simulink model "Drivetrain_Bicycle"  (R2020a)
settings: Solver=VariableStepAuto  StartTime=0.0  StopTime=10.0  RelTol=1e-3
settings Model: Creator=yafta  LastModifiedBy=yafta

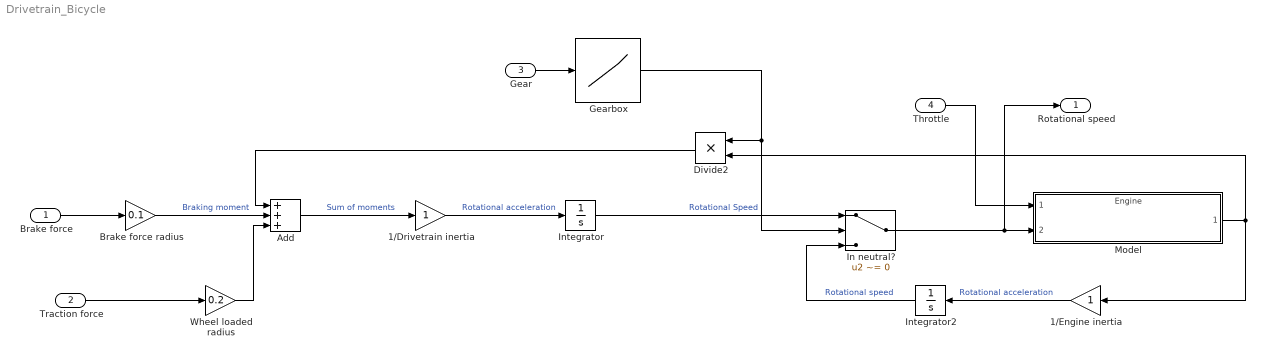
== system Drivetrain_Bicycle ==
  Brake force : Inport  OutDataTypeStr=double
  Traction force : Inport  Port=2  OutDataTypeStr=double
  Gear : Inport  Port=3  OutDataTypeStr=int8
  Throttle : Inport  Port=4  OutDataTypeStr=double
  1/Drivetrain inertia : Gain
  1/Engine inertia : Gain
  Add : Sum  Inputs=3
  Brake force radius : Gain  Gain=0.1
  Divide2 : Product  Inputs=**
  Gearbox : Lookup_n-D  NumberOfTableDimensions=1  BreakpointsForDimension1=[0,1,2,3,4,5,6]  BreakpointsForDimension1DataTypeStr=int8  Table=[0,2.583,2,1.667,1.444,1.286,1.15]  TableMin=0  TableMax=5  TableDataTypeStr=double  InterpMethod=Flat  DiagnosticForOutOfRangeInput=Error  InternalRulePriority=Speed  OutDataTypeStr=double  RndMeth=Simplest  InputSameDT=on
  In neutral? : Switch  Criteria=u2 ~= 0
  Integrator : Integrator
  Integrator2 : Integrator
  Model : ModelReference  ModelNameDialog=Engine  SimulationMode=Normal  ModelReferenceVersion=1.2
  Wheel loaded radius : Gain  Gain=0.2
  Rotational speed : Outport  OutDataTypeStr=double
  wires:
  1/Engine inertia/1 -> Integrator2/1  "Rotational acceleration"
  Traction force/1 -> Wheel loaded radius/1
  Integrator2/1 -> In neutral?/3  "Rotational speed"
  In neutral?/1 -> Model/2, Rotational speed/1
  Divide2/1 -> Add/1
  Integrator/1 -> In neutral?/1  "Rotational Speed"
  Brake force radius/1 -> Add/2  "Braking moment"
  Add/1 -> 1/Drivetrain inertia/1  "Sum of moments"
  Gearbox/1 -> In neutral?/2, Divide2/1
  Wheel loaded radius/1 -> Add/3
  Model/1 -> 1/Engine inertia/1, Divide2/2
  1/Drivetrain inertia/1 -> Integrator/1  "Rotational acceleration"
  Brake force/1 -> Brake force radius/1
  Gear/1 -> Gearbox/1
  Throttle/1 -> Model/1
